simulink subsystem "DC_Motor_armature"  (R2024b)
settings: Solver=VariableStepAuto  StartTime=0.0  StopTime=10.0  RelTol=1e-3
undefined symbols (not defined in the file or in its folder): DC
settings Model: Creator=Santiago  LastModifiedBy=SCK

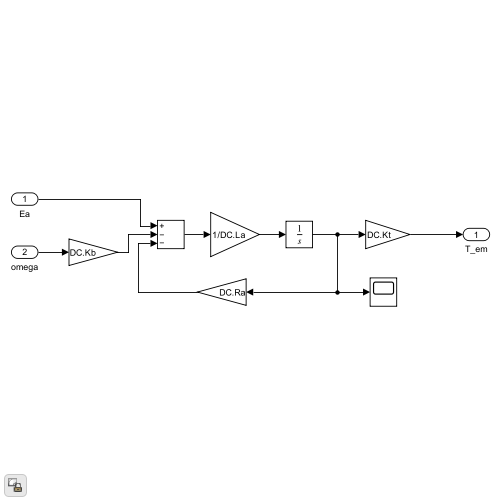
[thumbnail: Simulink's stored preview of the top-level diagram]
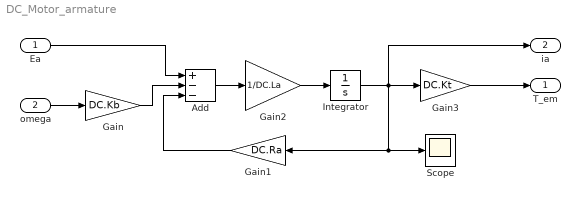
== system DC_Motor_armature ==
  Ea : Inport
  omega : Inport  Port=2
  Add : Sum  Inputs=+--
  Gain : Gain  Gain=DC.Kb
  Gain1 : Gain  Gain=DC.Ra
  Gain2 : Gain  Gain=1/DC.La
  Gain3 : Gain  Gain=DC.Kt
  Integrator : Integrator
  Scope : Scope
  T_em : Outport
  ia : Outport  Port=2
  wires:
  Gain3/1 -> T_em/1
  Ea/1 -> Add/1
  Integrator/1 -> Gain1/1, Scope/1, Gain3/1, ia/1
  omega/1 -> Gain/1
  Gain2/1 -> Integrator/1
  Gain1/1 -> Add/3
  Add/1 -> Gain2/1
  Gain/1 -> Add/2
